simulink model "StateMach"  (R2016a)
settings: Solver=FixedStepDiscrete  SolverMode=SingleTasking  StartTime=0.0  StopTime=20  FixedStep=0.001  RelTol=1e-3
settings Model: Creator=willi  LastModifiedBy=willi
settings OptimizationCC: DefaultParameterBehavior=Inlined  UseDivisionForNetSlopeComputation=on  UseFloatMulNetSlope=on  InlineInvariantSignals=on  PassReuseOutputArgsAs=Individual arguments  ZeroExternalMemoryAtStartup=off  ZeroInternalMemoryAtStartup=off  NoFixptDivByZeroProtection=on  EfficientFloat2IntCast=on  OptimizeModelRefInitCode=on  LifeSpan=1
settings HardwareCC: ProdBitPerPointer=32  ProdLargestAtomicInteger=Long  ProdLargestAtomicFloat=Double  ProdWordSize=32  ProdHWDeviceType=ARM Compatible->ARM Cortex
settings RTWCC: SystemTargetFile=ert.tlc  TemplateMakefile=ert_default_tmf  GenerateReport=on  IncludeHyperlinkInReport=on  LaunchReport=on  GenerateTraceInfo=on  GenerateTraceReport=on  GenerateTraceReportSl=on  GenerateTraceReportSf=on  GenerateTraceReportEml=on  GenerateCodeMetricsReport=on
settings CodeAppCC: ForceParamTrailComments=on  IgnoreCustomStorageClasses=off  OperatorAnnotations=on  SimulinkDataObjDesc=on  SFDataObjDesc=on  MATLABFcnDesc=on  CustomSymbolStrGlobalVar=rt$N$M  CustomSymbolStrType=$N$M  CustomSymbolStrFcn=$N$M$F  CustomSymbolStrMacro=$N$M  InsertBlockDesc=on  MATLABSourceComments=on
settings ERTTargetCC: GenerateSampleERTMain=on  IncludeMdlTerminateFcn=off  CombineSignalStateStructs=on  SupportAbsoluteTime=off  SupportComplex=off  PurelyIntegerCode=on  SupportNonInlinedSFcns=on  InlinedParameterPlacement=NonHierarchical  ERTCustomFileTemplate=example_file_process.tlc  ERTFilePackagingFormat=CompactWithDataFile

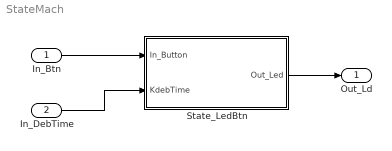
== system StateMach ==
  In_Btn : Inport  OutDataTypeStr=boolean  PortDimensions=1  Interpolate=off
  In_DebTime : Inport  Port=2  OutDataTypeStr=uint16  PortDimensions=1
  State_LedBtn : Stateflow chart  TreatAsAtomicUnit=on
  Out_Ld : Outport  OutDataTypeStr=boolean
  wires:
  State_LedBtn/1(Out_Led) -> Out_Ld/1
  In_Btn/1 -> State_LedBtn/1(In_Button)
  In_DebTime/1 -> State_LedBtn/2(KdebTime)

== stateflow chart StateMach/State_LedBtn ==
  state Led_Off
    entry:
    Out_Led = false;
  state Debounce
    entry:
    debTime = uint16(0.0);
    during:
    debTime = debTime + 1.0;
  state Led_On
    entry:
    Out_Led = true;
  (default) -> Led_Off
  Led_Off -> Debounce : [In_Button == true]
  Debounce -> Led_On [order 1] : [(debTime > KdebTime) && (In_Button == true)]
  Debounce -> Led_Off [order 2] : [(debTime > KdebTime) && (In_Button == false)]
  Led_On -> Debounce : [In_Button == false]
  data: In_Button input boolean size=1 [0..1]; Out_Led output boolean size=1 [0..1] =false; debTime local uint16; KdebTime input uint16
